simulink library "common_lib"  (R2023a)
settings: Solver=ode45  StartTime=0.0  StopTime=10.0  RelTol=1e-3
undefined symbols (not defined in the file): ACCEL_PRE_MULT, APDT_SrvcMgr_IRVHVDCSubFcnReq, C_C1GearNumbers, C_C1GearRatios, C_Calibration, C_DitherWaveform, C_GearOffset, C_GearRatioIn, C_GearRatioInverseOut, C_GearRatioOut, CLUTCH_INNER_LOOP_UPDATE_RATE, CONSTANT, DEGRADED_MODE_SIZE, Dem_EventStatusType, DiscIntNeverNeededParam, F_FAULT_ENUM, F_NOFAULT, F_OUTOFRANGE, F_RATELIMIT, FALSE, FMI14_SPECIAL_INSTRUCTIONS, FMI20_DATA_DRIFTED_HIGH, FMI21_DATA_DRIFTED_LOW, FMI29_RESERVED_FOR_SAE_ASSIGNMENT, FMI30_RESERVED_FOR_SAE_ASSIGNMENT, FMI31_CONDITION_EXISTS, FMI32_NO_FAULT, IC, k_accel, k_mean, MAX_UINT32, MEAN_PRE_MULT, NTriggers, QLTY_SIGNAL_FAILED, QLTY_SIGNAL_FULLY_FUNCTION, QLTY_SIGNAL_SUBSTITUTED_BY_1ST_CHOICE, QLTY_SIGNAL_SUBSTITUTED_BY_2ND_CHOICE, QLTY_SIGNAL_SUBSTITUTED_BY_3RD_CHOICE, QLTY_SIGNAL_SUBSTITUTED_BY_4TH_CHOICE, SAMPLE_TIME_100us, SAMPLETIME_10ms_Int, SATURATION_U16, simin, T_TestPoint, TF_FALSE, TF_TRUE, TimeStep, TRUE, WORKSPACE_UPDATE_RATE, ZERO, Zero
libraries: $bdroot x123, simulink x28, simulink_extras x4, MBD_EPS_Local_Blockset x4
(part 7 of 10)

== system common_lib/Gear Ratios/FindGearNumberByRatio ==
  note: If either the output speed, or the clutch speed is above minimum
      | then report that the speed is above minimum speed for detection.  However,
      | only output a gear other than zero to the GearNumber if OS > min speed.  This is done
      | because if the OS is stopped, but the clutch speed is still > min, you can tell
      | that there is no ratio being imposed.  So GearNumber should report zero, and the speeds are
      | above the threshold for detecting this condition.
  note: This block finds the gear number that corresponds to the ratio
      | between the os and clutch speed.  The output speed must be above the MinSpeed, and the ratio must be
      | within the SpeedTolerance for at least a time of ConfirmTime before OutputValid goes true.
      | If OutputValid is false then the GearNumber output does not have any meaning.
  OutputSpeed : Inport
  ClutchSpeed : Inport  Port=2
  SpeedTolerance : Inport  Port=3
  MinSpeed : Inport  Port=4
  Abs : Abs  ZeroCross=off  SaturateOnIntegerOverflow=off
  Abs1 : Abs  ZeroCross=off  SaturateOnIntegerOverflow=off
  Abs2 : Abs  ZeroCross=off  SaturateOnIntegerOverflow=off
  ClampAroundZero : $bdroot/Misc/ClampAroundZero  Tol=single(0.1)
      settings: AttributesFormatString=tol=%<Tol>
  Constant1 : Constant  Value=ConfirmTime
  Constant2 : Constant  Value=single(0)
  GearToRatio : Lookup  InputValues=GearToRatioIn  Table=GearToRatioOut  LookUpMeth=Use Input Nearest  SaturateOnIntegerOverflow=off
  Logical Operator : Logic  AllPortsSameDT=off
  Logical Operator1 : Logic  Operator=OR  AllPortsSameDT=off
  Product1 : Product  Inputs=/*  RndMeth=Zero
  Product2 : Product  Inputs=**  RndMeth=Zero
  RatioToGear : Lookup  InputValues=RatioToGearIn  Table=RatioToGearOut  LookUpMeth=Use Input Nearest  SaturateOnIntegerOverflow=off
  Relational Operator : RelationalOperator  Operator=<  ZeroCross=off  InputSameDT=off
  Relational Operator1 : RelationalOperator  Operator=>  ZeroCross=off  InputSameDT=off
  Relational Operator2 : RelationalOperator  Operator=>  ZeroCross=off  InputSameDT=off
  Sum : Sum  Inputs=-+
  Switch : Switch  Threshold=0.5  ZeroCross=off  SaturateOnIntegerOverflow=off  InputSameDT=off
  Timer1 : Subsystem  mask{TimeStep=0}
      mask prompts: TimeStep "Time Step (double)"
      mask help:
      | This block outputs a boolean true when In has been true
      | for at least the TiggerTime time.
  GearNumber : Outport  VectorParamsAs1DForOutWhenUnconnected=off
  OutputValid : Outport  Port=2  VectorParamsAs1DForOutWhenUnconnected=off
  SpeedAboveMin : Outport  Port=3  VectorParamsAs1DForOutWhenUnconnected=off
  wires:
  Relational Operator2/1 -> Logical Operator1/2
  Abs2/1 -> Relational Operator2/1
  Logical Operator1/1 -> SpeedAboveMin/1
  ClampAroundZero/1 -> Product1/1, Product2/2, Abs1/1
  Constant1/1 -> Timer1/2(TriggerTime)
  Timer1/1(Out) -> Switch/2, OutputValid/1
  Logical Operator/1 -> Timer1/1(In)
  Product1/1 -> RatioToGear/1
  ClutchSpeed/1 -> Abs2/1, Sum/2, Product1/2
  RatioToGear/1 -> GearToRatio/1, Switch/1  "nearest_gear_number"
  GearToRatio/1 -> Product2/1  "nearest_ratio"
  Product2/1 -> Sum/1  "nearest_speed_byratio"
  Abs/1 -> Relational Operator/1
  Sum/1 -> Abs/1
  SpeedTolerance/1 -> Relational Operator/2
  Relational Operator/1 -> Logical Operator/1
  Constant2/1 -> Switch/3
  OutputSpeed/1 -> ClampAroundZero/1
  Switch/1 -> GearNumber/1
  Abs1/1 -> Relational Operator1/1
  MinSpeed/1 -> Relational Operator2/2, Relational Operator1/2
  Relational Operator1/1 -> Logical Operator1/1, Logical Operator/2

== system common_lib/Gear Ratios/GearNumberToRatio ==
  gear_number : Inport
  C_GearInverseRatio : LookupNDDirect  NumberOfTableDimensions=1  Table=C_GearRatioInverseOut
  C_GearRatio : LookupNDDirect  NumberOfTableDimensions=1  Table=C_GearRatioOut
  Constant5 : Constant  Value=int8(-99)  SampleTime=-1
  GearOffset : Constant  Value=C_GearOffset  SampleTime=-1
  GearOffset1 : Constant  Value=int8(0)  SampleTime=-1
  Relational Operator3 : RelationalOperator  Operator=~=  ZeroCross=off
  Subtract : Sum
  Switch : Switch  Threshold=0.5  ZeroCross=off  SaturateOnIntegerOverflow=off  InputSameDT=off
  ratio : Outport  VectorParamsAs1DForOutWhenUnconnected=off
  inv_ratio : Outport  Port=2  VectorParamsAs1DForOutWhenUnconnected=off
  wires:
  GearOffset1/1 -> Switch/3
  Relational Operator3/1 -> Switch/2
  Constant5/1 -> Relational Operator3/2
  GearOffset/1 -> Subtract/2
  Subtract/1 -> C_GearRatio/1, C_GearInverseRatio/1
  Switch/1 -> Subtract/1
  gear_number/1 -> Switch/1, Relational Operator3/1
  C_GearRatio/1 -> ratio/1
  C_GearInverseRatio/1 -> inv_ratio/1

== system common_lib/IO/Calibration with Pretty Print Value ==
  C_Calibration : Constant  Value=CalValue  SampleTime=-1
  Outport : Outport  VectorParamsAs1DForOutWhenUnconnected=off
  wires:
  C_Calibration/1 -> Outport/1

== system common_lib/IO/From Workspace w//Datatype ==
  Data Type Conversion : DataTypeConversion  SaturateOnIntegerOverflow=off  RndMeth=Floor
  From Workspace : FromWorkspace  VariableName=var  SampleTime=st  ZeroCross=off
  Out1 : Outport  VectorParamsAs1DForOutWhenUnconnected=off
  wires:
  From Workspace/1 -> Data Type Conversion/1
  Data Type Conversion/1 -> Out1/1

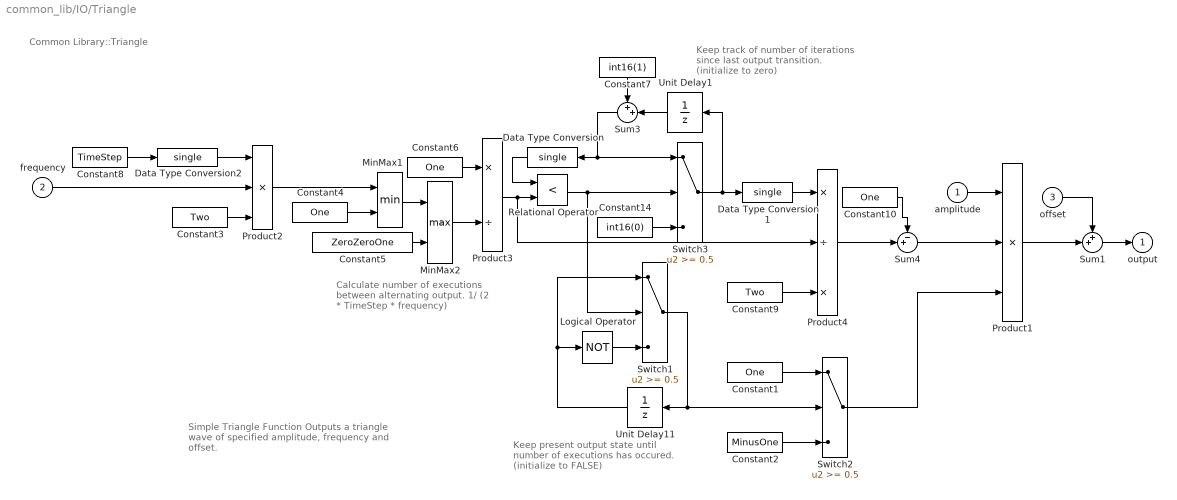
== system common_lib/IO/Triangle ==
  note: Common Library::Triangle
  note: Simple Triangle Function
      | Outputs a triangle wave of specified
      | amplitude, frequency and offset.
  note: Calculate number of executions
      | between alternating output.
      | 1/ (2 * TimeStep * frequency)
  note: Keep track of number of iterations
      | since last output transition.
      | (initialize to zero)
  note: Keep present output state until
      | number of executions has occured.
      | (initialize to FALSE)
  amplitude : Inport
  frequency : Inport  Port=2
  offset : Inport  Port=3
  Constant{1,4,6,10} (4 alike) : Constant  Value=One
  Constant14 : Constant  Value=int16(0)
  Constant2 : Constant  Value=MinusOne
  Constant3 : Constant  Value=Two
  Constant5 : Constant  Value=ZeroZeroOne
  Constant7 : Constant  Value=int16(1)
  Constant8 : Constant  Value=TimeStep
  Constant9 : Constant  Value=Two
  Data Type Conversion : DataTypeConversion  OutDataTypeStr=single  SaturateOnIntegerOverflow=off
  Data Type Conversion1 : DataTypeConversion  OutDataTypeStr=single  SaturateOnIntegerOverflow=off
  Data Type Conversion2 : DataTypeConversion  OutDataTypeStr=single  SaturateOnIntegerOverflow=off  RndMeth=Floor
  Logical Operator : Logic  Operator=NOT
  MinMax1 : MinMax  Inputs=2  InputSameDT=on  SaturateOnIntegerOverflow=on  ZeroCross=off
  MinMax2 : MinMax  Function=max  Inputs=2  InputSameDT=on  SaturateOnIntegerOverflow=on  ZeroCross=off
  Product1 : Product  Inputs=3  InputSameDT=on  OutDataTypeStr=Inherit: Same as first input
  Product2 : Product  Inputs=***  InputSameDT=on  OutDataTypeStr=Inherit: Same as first input
  Product3 : Product  Inputs=*/  InputSameDT=on  OutDataTypeStr=Inherit: Same as first input
  Product4 : Product  Inputs=*/*  InputSameDT=on  OutDataTypeStr=Inherit: Same as first input
  Relational Operator : RelationalOperator  Operator=<  ZeroCross=off
  Sum1 : Sum  Inputs=++|  InputSameDT=on  OutDataTypeStr=Inherit: Same as first input
  Sum3 : Sum  Inputs=++|  InputSameDT=on  OutDataTypeStr=Inherit: Same as first input
  Sum4 : Sum  Inputs=-+|  InputSameDT=on  OutDataTypeStr=Inherit: Same as first input
  Switch1 : Switch  Threshold=0.5  ZeroCross=off  SaturateOnIntegerOverflow=off
  Switch2 : Switch  Threshold=0.5  ZeroCross=off  SaturateOnIntegerOverflow=off
  Switch3 : Switch  Threshold=0.5  ZeroCross=off  SaturateOnIntegerOverflow=off
  Unit Delay1 : UnitDelay  SampleTime=-1  HasFrameUpgradeWarning=on
  Unit Delay11 : UnitDelay  InitialCondition=false  SampleTime=-1  HasFrameUpgradeWarning=on
  output : Outport  VectorParamsAs1DForOutWhenUnconnected=off
  wires:
  Constant8/1 -> Data Type Conversion2/1
  Data Type Conversion2/1 -> Product2/1
  Switch2/1 -> Product1/3
  Constant2/1 -> Switch2/3
  Constant1/1 -> Switch2/1
  Sum4/1 -> Product1/2
  Product4/1 -> Sum4/2
  Constant10/1 -> Sum4/1
  Constant9/1 -> Product4/3
  Data Type Conversion1/1 -> Product4/1
  offset/1 -> Sum1/1
  Unit Delay11/1 -> Logical Operator/1, Switch1/1
  Switch1/1 -> Switch2/2, Unit Delay11/1
  Product1/1 -> Sum1/2
  amplitude/1 -> Product1/1
  frequency/1 -> Product2/2
  Product2/1 -> MinMax1/1
  Constant4/1 -> MinMax1/2
  MinMax1/1 -> MinMax2/1
  Constant5/1 -> MinMax2/2
  Sum1/1 -> output/1
  MinMax2/1 -> Product3/2
  Constant6/1 -> Product3/1
  Constant3/1 -> Product2/3
  Switch3/1 -> Data Type Conversion1/1, Unit Delay1/1
  Constant14/1 -> Switch3/3
  Unit Delay1/1 -> Sum3/2
  Constant7/1 -> Sum3/1
  Sum3/1 -> Switch3/1, Data Type Conversion/1
  Logical Operator/1 -> Switch1/3
  Product3/1 -> Product4/2, Relational Operator/2
  Relational Operator/1 -> Switch3/2, Switch1/2
  Data Type Conversion/1 -> Relational Operator/1

== system common_lib/Integrators/ForwardEulerIntergrator ==
  dx : Inport
  x0 : Inport  Port=2
  reset : Inport  Port=3
  Constant2 : Constant  Value=TSAMP  SampleTime=-1
  Data Type Conversion : DataTypeConversion  OutDataTypeStr=single  SaturateOnIntegerOverflow=off
  Divide : Product  Inputs=**
  Sum : Sum  Inputs=|++
  Switch1 : Switch  Threshold=0.5  ZeroCross=off  SaturateOnIntegerOverflow=off  InputSameDT=off
  Unit Delay : UnitDelay  InitialCondition=IC  SampleTime=-1  HasFrameUpgradeWarning=on
      settings: AttributesFormatString=ic=%<X0>
  x : Outport  VectorParamsAs1DForOutWhenUnconnected=off
  wires:
  Data Type Conversion/1 -> Divide/2
  Sum/1 -> Unit Delay/1
  Unit Delay/1 -> Switch1/3
  Switch1/1 -> x/1, Sum/2
  x0/1 -> Switch1/1
  reset/1 -> Switch1/2
  dx/1 -> Divide/1
  Divide/1 -> Sum/1
  Constant2/1 -> Data Type Conversion/1

== system common_lib/Misc/ArcSine ==
  note: Common Library::Trigonometry:Sine
  note: Taylor Series Expansion for ArcSIN
      | Best Accuracy from -pi/3 to +pi/3
  angle : Inport
  Constant5 : Constant  Value=single(1/6)
  Constant6 : Constant  Value=single(3/40)
  Constant7 : Constant  Value=single(15/336)
  Constant9 : Constant  Value=single(105/3456)
  Product{1..2,4..5} (4 alike) : Product  OutDataTypeStr=Inherit: Same as first input
  Product{3,6..8} (4 alike) : Product  Inputs=3  OutDataTypeStr=Inherit: Same as first input
  Sum1 : Sum  Inputs=5
  asin : Outport  VectorParamsAs1DForOutWhenUnconnected=off
  wires:
  Sum1/1 -> asin/1
  Product6/1 -> Product4/1
  Product4/1 -> Sum1/5
  angle/1 -> Product7/2, Sum1/1, Product8/1, Product8/2, Product8/3, Product7/3, Product3/2, Product3/3, Product6/3, Product6/2
  Constant9/1 -> Product4/2
  Product2/1 -> Sum1/4
  Constant7/1 -> Product2/2
  Product3/1 -> Product2/1, Product6/1
  Product1/1 -> Sum1/3
  Constant6/1 -> Product1/2
  Product7/1 -> Product1/1, Product3/1
  Product5/1 -> Sum1/2
  Constant5/1 -> Product5/2
  Product8/1 -> Product7/1, Product5/1

== system common_lib/Misc/ClampAboveZero ==
  note: Common Library::Miscellaneous Computations::Clamp Above Zero
  input : Inport
  Constant : Constant  Value=Tol
  MinMax : MinMax  Function=max  Inputs=2  InputSameDT=on  SaturateOnIntegerOverflow=on  ZeroCross=off
  output : Outport  VectorParamsAs1DForOutWhenUnconnected=off
  wires:
  input/1 -> MinMax/1
  MinMax/1 -> output/1
  Constant/1 -> MinMax/2

== system common_lib/Misc/ClampAroundZero ==
  note: Common Library::Miscellaneous Computations::Clamp Around Zero
  input : Inport
  Abs : Abs  ZeroCross=off  SaturateOnIntegerOverflow=off
  Constant : Constant  Value=Tol
  Constant1 : Constant  Value=Zero
  Constant2 : Constant  Value=One
  Constant3 : Constant  Value=MinusOne
  MinMax : MinMax  Function=max  Inputs=2  InputSameDT=on  SaturateOnIntegerOverflow=on  ZeroCross=off
  Product : Product  InputSameDT=on  OutDataTypeStr=Inherit: Same as first input
  Relational Operator : RelationalOperator  ZeroCross=off
  Switch1 : Switch  Threshold=0.5  ZeroCross=off  SaturateOnIntegerOverflow=off
  output : Outport  VectorParamsAs1DForOutWhenUnconnected=off
  wires:
  Constant/1 -> MinMax/2
  Abs/1 -> MinMax/1
  input/1 -> Abs/1, Relational Operator/1
  MinMax/1 -> Product/2
  Switch1/1 -> Product/1
  Product/1 -> output/1
  Constant1/1 -> Relational Operator/2
  Relational Operator/1 -> Switch1/2
  Constant2/1 -> Switch1/1
  Constant3/1 -> Switch1/3

== system common_lib/Misc/Cosine ==
  note: Taylor Series Expansion for COS(x)
  note: Common Library::Trigonometry:Cosine
  angle : Inport
  Constant : Constant  Value=single(1/(1*2))
  Constant1 : Constant  Value=single(1/(1*2*3*4))
  Constant2 : Constant  Value=single(1)
  Product : Product  OutDataTypeStr=Inherit: Same as first input
  Product1 : Product  OutDataTypeStr=Inherit: Same as first input
  Product3 : Product  OutDataTypeStr=Inherit: Same as first input
  Product6 : Product  Inputs=3  OutDataTypeStr=Inherit: Same as first input
  Sum : Sum  Inputs=+-+
  cos : Outport  VectorParamsAs1DForOutWhenUnconnected=off
  wires:
  Product/1 -> Sum/2
  Product1/1 -> Sum/3
  Sum/1 -> cos/1
  angle/1 -> Product3/2, Product6/2, Product6/3, Product3/1
  Product3/1 -> Product6/1, Product/1
  Constant1/1 -> Product1/2
  Constant/1 -> Product/2
  Product6/1 -> Product1/1
  Constant2/1 -> Sum/1

== system common_lib/Misc/Count Edges ==
  note: Common Library::Miscellaneous::Count Edges
  Input : Inport
  Reset : Inport  Port=2
  Logical Operator5 : Logic  Operator=NOT  AllPortsSameDT=off
  Logical Operator6 : Logic  AllPortsSameDT=off
  Sum : Sum  Inputs=|++  InputSameDT=on  OutDataTypeStr=Inherit: Same as first input
  Switch1 : Switch  Threshold=0.5  ZeroCross=off  SaturateOnIntegerOverflow=off  InputSameDT=off
  Switch2 : Switch  Threshold=0.5  ZeroCross=off  SaturateOnIntegerOverflow=off  InputSameDT=off
  Unit Delay2 : UnitDelay  InitialCondition=int8(0)  SampleTime=-1  HasFrameUpgradeWarning=on
      settings: AttributesFormatString=ic=%<X0>
  Unit Delay3 : UnitDelay  InitialCondition=true  SampleTime=-1  HasFrameUpgradeWarning=on
      settings: AttributesFormatString=ic=%<X0>
  constant7 : Constant  Value=int8(0)
  constant8 : Constant  Value=int8(1)
  constant9 : Constant  Value=int8(0)
  Count : Outport  VectorParamsAs1DForOutWhenUnconnected=off
  wires:
  Reset/1 -> Switch1/2
  Input/1 -> Logical Operator6/1, Unit Delay3/1
  Switch1/1 -> Sum/2
  Unit Delay2/1 -> Count/1, Switch1/3
  constant9/1 -> Switch1/1
  Switch2/1 -> Sum/1
  Logical Operator6/1 -> Switch2/2
  Logical Operator5/1 -> Logical Operator6/2
  Unit Delay3/1 -> Logical Operator5/1
  constant8/1 -> Switch2/1
  constant7/1 -> Switch2/3
  Sum/1 -> Unit Delay2/1

== system common_lib/Misc/Count to X ==
  note: Common Library::Miscellaneous::Count to X
  input : Inport
  reset? : Inport  Port=2
  Constant1 : Constant  Value=uint8(1)
  Constant2 : Constant  Value=uint8(0)
  Constant3 : Constant  Value=uint8(X)
  Constant4 : Constant  Value=uint8(0)
  DelayedInput : Logic  Operator=NAND
  Input : Logic
  Logical Operator8 : Logic
  MinMax : MinMax  Inputs=2  InputSameDT=on  SaturateOnIntegerOverflow=on  ZeroCross=off
  Relational Operator : RelationalOperator  ZeroCross=off
  Sum1 : Sum  Inputs=++|  InputSameDT=on  OutDataTypeStr=Inherit: Same as first input
  Unit Delay : UnitDelay  InitialCondition=uint8(0)  SampleTime=-1  HasFrameUpgradeWarning=on
  Unit Delay2 : UnitDelay  InitialCondition=false  SampleTime=-1  HasFrameUpgradeWarning=on
  inc switch : Switch  Threshold=0.5  ZeroCross=off  SaturateOnIntegerOverflow=off
  reset switch : Switch  Threshold=0.5  ZeroCross=off  SaturateOnIntegerOverflow=off
  output : Outport  VectorParamsAs1DForOutWhenUnconnected=off
  wires:
  Relational Operator/1 -> output/1
  Constant3/1 -> Relational Operator/2, MinMax/1
  Constant2/1 -> inc switch/3
  Constant1/1 -> inc switch/1
  Constant4/1 -> reset switch/1
  input/1 -> Unit Delay2/1, Input/1, Input/2
  Input/1 -> Logical Operator8/1
  Unit Delay2/1 -> DelayedInput/1, DelayedInput/2
  DelayedInput/1 -> Logical Operator8/2
  inc switch/1 -> Sum1/2
  Logical Operator8/1 -> inc switch/2
  Sum1/1 -> Relational Operator/1, MinMax/2
  reset switch/1 -> Sum1/1
  Unit Delay/1 -> reset switch/3
  reset?/1 -> reset switch/2
  MinMax/1 -> Unit Delay/1

== system common_lib/Misc/Counter ==
  note: Counter increments when "incr condition" is TRUE and decrements when "decr condition" is TRUE.
  note: Common Library::Miscellaneous::Counter
  up_val : Inport
  count_up? : Inport  Port=2  OutDataTypeStr=boolean
  down_val : Inport  Port=3
  count_down? : Inport  Port=4  OutDataTypeStr=boolean
  max_count : Inport  Port=5
  min_count : Inport  Port=6
  reset? : Inport  Port=7  OutDataTypeStr=boolean
  Constant1 : Constant  Value=Zero
  Constant2 : Constant  Value=Zero
  Constant4 : Constant  Value=IC
  Constant5 : Constant  Value=false
  Logical Operator : Logic  Operator=OR
  Sat : $bdroot/Slink/Sat
  Sum : Sum  Inputs=++-  InputSameDT=on  OutDataTypeStr=Inherit: Same as first input
  Unit Delay : UnitDelay  InitialCondition=IC  SampleTime=-1  HasFrameUpgradeWarning=on
  Unit Delay1 : UnitDelay  InitialCondition=true  SampleTime=-1  HasFrameUpgradeWarning=on
  dec switch : Switch  Threshold=0.5  ZeroCross=off  SaturateOnIntegerOverflow=off
  inc switch : Switch  Threshold=0.5  ZeroCross=off  SaturateOnIntegerOverflow=off
  reset switch : Switch  Threshold=0.5  ZeroCross=off  SaturateOnIntegerOverflow=off
  output : Outport  VectorParamsAs1DForOutWhenUnconnected=off
  wires:
  count_down?/1 -> dec switch/2
  down_val/1 -> dec switch/1
  count_up?/1 -> inc switch/2
  up_val/1 -> inc switch/1
  Constant2/1 -> dec switch/3
  dec switch/1 -> Sum/3
  Constant1/1 -> inc switch/3
  inc switch/1 -> Sum/2
  reset?/1 -> Logical Operator/1
  reset switch/1 -> Unit Delay/1, output/1
  Unit Delay/1 -> Sum/1
  Logical Operator/1 -> reset switch/2
  Unit Delay1/1 -> Logical Operator/2
  Constant5/1 -> Unit Delay1/1
  Sat/1 -> reset switch/3
  Constant4/1 -> reset switch/1
  max_count/1 -> Sat/2
  min_count/1 -> Sat/3
  Sum/1 -> Sat/1

== system common_lib/Misc/Divide by X ==
  note: Common Library::Miscellaneous::Divide by X
  trigger? : Inport
  Constant1 : Constant  Value=uint8(X)
  Constant2 : Constant  Value=uint8(1)
  Constant3 : Constant  Value=uint8(X)
  Constant4 : Constant  Value=uint8(0)
  Relational Operator : RelationalOperator  ZeroCross=off
  Sum1 : Sum  Inputs=|++  InputSameDT=on  OutDataTypeStr=Inherit: Same as first input
  Unit Delay : UnitDelay  InitialCondition=uint8(X)  SampleTime=-1  HasFrameUpgradeWarning=on
  inc switch : Switch  Threshold=0.5  ZeroCross=off  SaturateOnIntegerOverflow=off
  reset switch : Switch  Threshold=0.5  ZeroCross=off  SaturateOnIntegerOverflow=off
  output : Outport  VectorParamsAs1DForOutWhenUnconnected=off
  wires:
  Constant4/1 -> reset switch/1
  Constant1/1 -> inc switch/1
  Constant2/1 -> Sum1/1
  trigger?/1 -> inc switch/2
  Sum1/1 -> inc switch/3
  inc switch/1 -> Relational Operator/1, reset switch/3
  Constant3/1 -> Relational Operator/2
  Unit Delay/1 -> Sum1/2
  Relational Operator/1 -> reset switch/2, output/1
  reset switch/1 -> Unit Delay/1

== system common_lib/Misc/EatonLogo ==

== system common_lib/Misc/EdgeTriggered Pulse ==
  note: Common Library::Miscellaneous::Edge Triggered Pulse
  input : Inport
  ETP : $bdroot/Misc/EdgeTriggered Pulse w time  Edge=TRUE to FALSE  Pulse=TRUE  TimeStep=[]  Init=0
  Timeout Threshold : Constant  Value=Width
  pulse : Outport  VectorParamsAs1DForOutWhenUnconnected=off
  wires:
  input/1 -> ETP/1
  Timeout Threshold/1 -> ETP/2
  ETP/1 -> pulse/1

== system common_lib/Misc/EdgeTriggered Pulse w time ==
  note: 0 = PULSE_FALSE
      | 1 = PULSE_TRUE
  note: 0 = FALSE_TO_TRUE
      | 1 = TRUE_TO_FALSE
  input : Inport  OutDataTypeStr=boolean
  width : Inport  Port=2  OutDataTypeStr=single
  Data Type Conversion : DataTypeConversion  OutDataTypeStr=single  RndMeth=Floor
  EdgeTriggeredPulseCoreLogic : Subsystem  TreatAsAtomicUnit=on  RTWFcnName=ETPWT
      settings: RTWSystemCode=Inline  RTWFcnNameOpts=User specified  RTWFileNameOpts=Use function name
  Output : Constant  Value=OUTPUT
  Trigger : Constant  Value=TRIGGER
  XOR_IN : Logic  Operator=XOR
  XOR_OUT : Logic  Operator=XOR
  pulse : Outport  OutDataTypeStr=boolean  VectorParamsAs1DForOutWhenUnconnected=off
  wires:
  XOR_IN/1 -> EdgeTriggeredPulseCoreLogic/1(input)
  width/1 -> Data Type Conversion/1
  Output/1 -> XOR_OUT/1
  EdgeTriggeredPulseCoreLogic/1(pulse) -> XOR_OUT/2
  XOR_OUT/1 -> pulse/1
  input/1 -> XOR_IN/2
  Trigger/1 -> XOR_IN/1
  Data Type Conversion/1 -> EdgeTriggeredPulseCoreLogic/2(width)

== system common_lib/Misc/GreenLeaf_Globe ==

== system common_lib/Misc/Hold ==
  in : Inport
  Enable : EnablePort  ZeroCross=off
  out : Outport  VectorParamsAs1DForOutWhenUnconnected=off
  wires:
  in/1 -> out/1

== system common_lib/Misc/Latch ==
  note: Output signal is latched to true until reset input is true.
  note: Common Library::Miscellaneous::Latch
  input : Inport  OutDataTypeStr=boolean
  reset? : Inport  Port=2  OutDataTypeStr=boolean
  Constant2 : Constant  Value=false
  Constant3 : Constant  Value=true
  Switch : Switch  Threshold=0.5  ZeroCross=off
  Switch1 : Switch  Threshold=0.5  ZeroCross=off
  Unit Delay1 : UnitDelay  InitialCondition=IC  SampleTime=-1  HasFrameUpgradeWarning=on
  output : Outport  VectorParamsAs1DForOutWhenUnconnected=off
  wires:
  Switch/1 -> Unit Delay1/1, output/1
  reset?/1 -> Switch/2
  Constant2/1 -> Switch/1
  Switch1/1 -> Switch/3
  Unit Delay1/1 -> Switch1/3
  input/1 -> Switch1/2
  Constant3/1 -> Switch1/1

== system common_lib/Misc/ModelVersion ==
  Terminator : Terminator
  mdlVersionBlock : Constant  Value=mdlVersion  SampleTime=-1
  wires:
  mdlVersionBlock/1 -> Terminator/1  "DiagBusVolt_SwcVer"

== system common_lib/Misc/NonZero ==
  InputValue : Inport
  Abs : Abs  ZeroCross=off
  Constant : Constant  Value=Tol
  Relational Operator : RelationalOperator  ZeroCross=off  InputSameDT=off
  SrvcMgr_IGBTSrvcIGBT6Offset : Outport  InitialOutput=APDT_SrvcMgr_IRVHVDCSubFcnReq.SrvcMgr_IRVHVDCSubFcnReq_NoReq  VectorParamsAs1DForOutWhenUnconnected=off
  wires:
  InputValue/1 -> Abs/1
  Relational Operator/1 -> SrvcMgr_IGBTSrvcIGBT6Offset/1
  Constant/1 -> Relational Operator/2
  Abs/1 -> Relational Operator/1

== system common_lib/Misc/Sine ==
  note: Taylor Series Expansion for SIN(x)
  note: Common Library::Trigonometry:Sine
  angle : Inport
  Constant : Constant  Value=single(1/(1*2*3))
  Constant1 : Constant  Value=single(1/(1*2*3*4*5))
  Product : Product  OutDataTypeStr=Inherit: Same as first input
  Product1 : Product  OutDataTypeStr=Inherit: Same as first input
  Product3 : Product  Inputs=3  OutDataTypeStr=Inherit: Same as first input
  Product6 : Product  Inputs=3  OutDataTypeStr=Inherit: Same as first input
  Sum : Sum  Inputs=+-+
  sin : Outport  VectorParamsAs1DForOutWhenUnconnected=off
  wires:
  Product/1 -> Sum/2
  Product1/1 -> Sum/3
  Sum/1 -> sin/1
  angle/1 -> Product6/3, Product6/2, Product3/3, Product3/2, Product3/1, Sum/1
  Product3/1 -> Product6/1, Product/1
  Constant1/1 -> Product1/2
  Constant/1 -> Product/2
  Product6/1 -> Product1/1

== system common_lib/Misc/Tangent ==
  note: Taylor Series Expansion for TAN(x)
  note: Common Library::Trigonometry::Tangent
  angle : Inport
  Constant : Constant  Value=single(1/3)
  Constant1 : Constant  Value=single(2/15)
  Product1 : Product  Inputs=3  OutDataTypeStr=Inherit: Same as first input
  Product3 : Product  OutDataTypeStr=Inherit: Same as first input
  Product4 : Product  OutDataTypeStr=Inherit: Same as first input
  Product6 : Product  Inputs=3  OutDataTypeStr=Inherit: Same as first input
  Sum : Sum  Inputs=+++
  tan : Outport  VectorParamsAs1DForOutWhenUnconnected=off
  wires:
  Product4/1 -> Sum/3
  Product3/1 -> Sum/2
  Constant/1 -> Product3/2
  angle/1 -> Sum/1, Product1/1, Product1/2, Product1/3, Product6/2, Product6/3
  Sum/1 -> tan/1
  Constant1/1 -> Product4/2
  Product1/1 -> Product3/1, Product6/1
  Product6/1 -> Product4/1

== system common_lib/Misc/Timeout Detection ==
  note: Common Library::Miscellaneous::Timeout Detection
  value : Inport
  Data Type Conversion : DataTypeConversion  OutDataTypeStr=single  SaturateOnIntegerOverflow=off  RndMeth=Floor
  Relational Operator : RelationalOperator  Operator===  OutDataTypeStr=boolean  ZeroCross=off
  Relational Operator1 : RelationalOperator  Operator=>  OutDataTypeStr=boolean  ZeroCross=off
  Timeout Threshold : Constant  Value=Timeout
  TimeoutLogic : Subsystem  TreatAsAtomicUnit=on  RTWFcnName=TIMEOUT
      settings: RTWSystemCode=Inline  RTWFcnNameOpts=User specified  RTWFileNameOpts=Use function name
  Unit Delay1 : UnitDelay  InitialCondition=Zero  SampleTime=-1  HasFrameUpgradeWarning=on
  timeout? : Outport  VectorParamsAs1DForOutWhenUnconnected=off
  wires:
  TimeoutLogic/1(time) -> Relational Operator1/1
  Timeout Threshold/1 -> Data Type Conversion/1
  Relational Operator1/1 -> timeout?/1
  Unit Delay1/1 -> Relational Operator/2
  Relational Operator/1 -> TimeoutLogic/1(Change)
  value/1 -> Unit Delay1/1, Relational Operator/1
  Data Type Conversion/1 -> Relational Operator1/2, TimeoutLogic/2(Timeout)

== system common_lib/Misc/Timeout with time ==
  note: Common Library::Miscellaneous::Timeout Detection
  value : Inport
  timeout : Inport  Port=2
  Data Type Conversion : DataTypeConversion  OutDataTypeStr=single  RndMeth=Floor
  Relational Operator : RelationalOperator  Operator===  OutDataTypeStr=boolean  ZeroCross=off
  Relational Operator1 : RelationalOperator  Operator=>  OutDataTypeStr=boolean  ZeroCross=off
  TimeoutLogic : Subsystem  TreatAsAtomicUnit=on  RTWFcnName=TIMEOUT
      settings: RTWSystemCode=Inline  RTWFcnNameOpts=User specified  RTWFileNameOpts=Use function name
  Unit Delay1 : UnitDelay  InitialCondition=Zero  SampleTime=-1  HasFrameUpgradeWarning=on
  timeout? : Outport  VectorParamsAs1DForOutWhenUnconnected=off
  wires:
  Data Type Conversion/1 -> TimeoutLogic/2(Timeout), Relational Operator1/2
  value/1 -> Relational Operator/1, Unit Delay1/1
  Relational Operator/1 -> TimeoutLogic/1(Change)
  Unit Delay1/1 -> Relational Operator/2
  Relational Operator1/1 -> timeout?/1
  timeout/1 -> Data Type Conversion/1
  TimeoutLogic/1(time) -> Relational Operator1/1

== system common_lib/Misc/Timeout with time Integer ==
  note: Common Library::Miscellaneous::Timeout Detection
  value : Inport
  timeout : Inport  Port=2
  Relational Operator : RelationalOperator  Operator===  OutDataTypeStr=boolean  ZeroCross=off
  Relational Operator1 : RelationalOperator  Operator=>  OutDataTypeStr=boolean  ZeroCross=off
  TimeoutLogic : Subsystem  TreatAsAtomicUnit=on  RTWFcnName=TIMEOUT
      settings: RTWSystemCode=Inline  RTWFcnNameOpts=User specified  RTWFileNameOpts=Use function name
  Unit Delay1 : UnitDelay  InitialCondition=Zero  SampleTime=-1  HasFrameUpgradeWarning=on
  timeout? : Outport  VectorParamsAs1DForOutWhenUnconnected=off
  wires:
  TimeoutLogic/1(time) -> Relational Operator1/1
  Relational Operator1/1 -> timeout?/1
  Unit Delay1/1 -> Relational Operator/2
  Relational Operator/1 -> TimeoutLogic/1(Change)
  value/1 -> Unit Delay1/1, Relational Operator/1
  timeout/1 -> Relational Operator1/2, TimeoutLogic/2(Timeout)

== system common_lib/Misc/Value Latch1 ==
  note: Common Library::Miscellaneous::Latch
  input : Inport
  Switch : Switch  Threshold=0.5  ZeroCross=off  SaturateOnIntegerOverflow=off
  Timeout Detection : $bdroot/Misc/Timeout Detection  Timeout=HoldTime  TimeStep=TimeStep
  Unit Delay : UnitDelay  InitialCondition=IC  SampleTime=-1  HasFrameUpgradeWarning=on
      settings: AttributesFormatString=ic=%<X0>
  Unit Delay1 : UnitDelay  InitialCondition=TRUE  SampleTime=-1  HasFrameUpgradeWarning=on
      settings: AttributesFormatString=ic=%<X0>
  output : Outport  InitialOutput=0  VectorParamsAs1DForOutWhenUnconnected=off
  wires:
  Unit Delay1/1 -> Timeout Detection/1
  Timeout Detection/1 -> Switch/2, Unit Delay1/1
  Unit Delay/1 -> Switch/3
  input/1 -> Switch/1
  Switch/1 -> Unit Delay/1, output/1

== system common_lib/OS/Scheduler ==
  Interrupt : TriggerPort  TriggerType=function-call  VariantControl=(inherit)  StatesWhenEnabling=reset  ZeroCross=off
  Demux : Demux  Outputs=5
      settings: DisplayOption=none
  Function-Call Generator : simulink/Ports & Subsystems/Function-Call Generator  sample_time=-1  numberOfIterations=1  DisallowWideOutput=off
  Task 1 : Outport  VectorParamsAs1DForOutWhenUnconnected=off
  Task 2 : Outport  Port=2  VectorParamsAs1DForOutWhenUnconnected=off
  Task 3 : Outport  Port=3  VectorParamsAs1DForOutWhenUnconnected=off
  Task 4 : Outport  Port=4  VectorParamsAs1DForOutWhenUnconnected=off
  Task 5 : Outport  Port=5  VectorParamsAs1DForOutWhenUnconnected=off
  wires:
  Function-Call Generator/1 -> Demux/1
  Demux/1 -> Task 1/1
  Demux/2 -> Task 2/1
  Demux/3 -> Task 3/1
  Demux/4 -> Task 4/1
  Demux/5 -> Task 5/1

== system common_lib/OS/Scheduler with Init ==
  Interrupt : TriggerPort  TriggerType=function-call  VariantControl=(inherit)  StatesWhenEnabling=reset  ZeroCross=off
  Demux : Demux  Outputs=3
      settings: DisplayOption=none
  Function-Call Generator : simulink/Ports & Subsystems/Function-Call Generator  sample_time=-1  numberOfIterations=1  DisallowWideOutput=off
  Init Relay : Subsystem
  Init : Outport  VectorParamsAs1DForOutWhenUnconnected=off
  Task 1 : Outport  Port=2  VectorParamsAs1DForOutWhenUnconnected=off
  Task 2 : Outport  Port=3  VectorParamsAs1DForOutWhenUnconnected=off
  wires:
  Demux/3 -> Task 2/1
  Demux/2 -> Task 1/1
  Demux/1 -> Init Relay/Trigger
  Init Relay/1(Init) -> Init/1
  Function-Call Generator/1 -> Demux/1

== system common_lib/OS/fcn_call generator ==
  note: This component is an atomic element used by the
      | schedule_morph script to build scheduler blocks
  note: Common Library::OS::Function Call Generator
  Enable : EnablePort  StatesWhenEnabling=reset  ZeroCross=off
  Function-Call Generator : simulink/Ports & Subsystems/Function-Call Generator  sample_time=-1  numberOfIterations=1  DisallowWideOutput=off
  Out : Outport  VectorParamsAs1DForOutWhenUnconnected=off
  wires:
  Function-Call Generator/1 -> Out/1

== system common_lib/OS/schedule counter ==
  note: This component is an atomic element used by the
      | schedule_morph script to build scheduler blocks
  note: Common Library::OS::Schedule Counter
  Constant2 : Constant  Value=int8(1)
  Constant3 : Constant  Value=int8(1)
  Constant4 : Constant  Value=FALSE
  Constant5 : Constant  Value=int8(1)
  Logical Operator : Logic  Operator=OR
  MinMax1 : MinMax  Inputs=2  InputSameDT=on  ZeroCross=off
  NTriggers : Constant  Value=NTriggers
  Relational Operator1 : RelationalOperator  Operator=>  ZeroCross=off  InputSameDT=off
  Sum : Sum  Inputs=++|  InputSameDT=on  OutDataTypeStr=Inherit: Same as first input
  Sum1 : Sum  Inputs=|-+  InputSameDT=on  OutDataTypeStr=Inherit: Same as first input
  Unit Delay : UnitDelay  InitialCondition=int8(1)  SampleTime=-1  HasFrameUpgradeWarning=on
  Unit Delay1 : UnitDelay  InitialCondition=TRUE  SampleTime=-1  HasFrameUpgradeWarning=on
  reset switch : Switch  Threshold=0.5  ZeroCross=off  SaturateOnIntegerOverflow=off
  Counter : Outport  VectorParamsAs1DForOutWhenUnconnected=off
  wires:
  Constant5/1 -> Sum1/1
  Sum/1 -> MinMax1/2
  NTriggers/1 -> Sum1/2, MinMax1/1
  Sum1/1 -> Relational Operator1/2
  Relational Operator1/1 -> Logical Operator/1
  Constant3/1 -> reset switch/1
  MinMax1/1 -> reset switch/3
  Constant2/1 -> Sum/2
  Constant4/1 -> Unit Delay1/1
  Unit Delay1/1 -> Logical Operator/2
  Logical Operator/1 -> reset switch/2
  Unit Delay/1 -> Relational Operator1/1, Sum/1
  reset switch/1 -> Unit Delay/1, Counter/1

== system common_lib/OS/sequence generator ==
  note: This component is an atomic element used by the
      | schedule_morph script to build scheduler blocks
  note: Common Library::OS::Sequence Generator
  In : Inport
  Constant9 : Constant  Value=int8(1)
  Function-Call Generator : simulink/Ports & Subsystems/Function-Call Generator  sample_time=-1  numberOfIterations=1  DisallowWideOutput=off
  Sum1 : Sum  Inputs=|++  InputSameDT=on  OutDataTypeStr=Inherit: Same as first input
  Trigger : Outport  VectorParamsAs1DForOutWhenUnconnected=off
  Out : Outport  Port=2  VectorParamsAs1DForOutWhenUnconnected=off
  wires:
  Function-Call Generator/1 -> Trigger/1
  Constant9/1 -> Sum1/2
  In/1 -> Sum1/1
  Sum1/1 -> Out/1

== system common_lib/SCond/Gain and Offset (in) ==
  note: Common Library::Signal Conditioning::Gain and Offset (in)
  input : Inport
  gain : Inport  Port=2
  offset : Inport  Port=3
  InputConversion : DataTypeConversion  OutDataTypeStr=single  SaturateOnIntegerOverflow=off
  InputConversion1 : DataTypeConversion  OutDataTypeStr=single  SaturateOnIntegerOverflow=off
  InputConversion2 : DataTypeConversion  OutDataTypeStr=single  SaturateOnIntegerOverflow=off
  OutputConversion : DataTypeConversion  OutDataTypeStr=single  SaturateOnIntegerOverflow=off
  Product : Product  InputSameDT=on  OutDataTypeStr=Inherit: Same as first input
  Sum : Sum  Inputs=|+-  InputSameDT=on  OutDataTypeStr=Inherit: Same as first input
  output : Outport  VectorParamsAs1DForOutWhenUnconnected=off
  wires:
  OutputConversion/1 -> output/1
  input/1 -> InputConversion/1
  gain/1 -> InputConversion1/1
  Product/1 -> Sum/1
  offset/1 -> InputConversion2/1
  Sum/1 -> OutputConversion/1
  InputConversion/1 -> Product/1
  InputConversion1/1 -> Product/2
  InputConversion2/1 -> Sum/2

== system common_lib/SCond/Gain and Offset (out) ==
  note: Common Library::Signal Conditioning::Gain and Offset (out)
  input : Inport
  gain : Inport  Port=2
  offset : Inport  Port=3
  InputConversion : DataTypeConversion  OutDataTypeStr=single  SaturateOnIntegerOverflow=off
  InputConversion1 : DataTypeConversion  OutDataTypeStr=single  SaturateOnIntegerOverflow=off
  InputConversion2 : DataTypeConversion  OutDataTypeStr=single  SaturateOnIntegerOverflow=off
  OutputConversion : DataTypeConversion  OutDataTypeStr=single  SaturateOnIntegerOverflow=off
  Product : Product  Inputs=*/  InputSameDT=on  OutDataTypeStr=Inherit: Same as first input
  Sum : Sum  Inputs=|++  InputSameDT=on  OutDataTypeStr=Inherit: Same as first input
  output : Outport  VectorParamsAs1DForOutWhenUnconnected=off
  wires:
  Sum/1 -> Product/1
  input/1 -> InputConversion/1
  OutputConversion/1 -> output/1
  offset/1 -> InputConversion1/1
  gain/1 -> InputConversion2/1
  Product/1 -> OutputConversion/1
  InputConversion/1 -> Sum/1
  InputConversion1/1 -> Sum/2
  InputConversion2/1 -> Product/2

== system common_lib/SCond/Membership Function ==
  x : Inport
  Compare1 : RelationalOperator  Operator=<=  ZeroCross=off
  MinMax : MinMax  Function=max  Inputs=2  InputSameDT=on  SaturateOnIntegerOverflow=on  ZeroCross=off
  Product2 : Product  Inputs=**  OutDataTypeStr=Inherit: Same as first input
  Sum1 : Sum  Inputs=|++  InputSameDT=on  OutDataTypeStr=Inherit: Same as first input
  Sum2 : Sum  Inputs=-+|  InputSameDT=on  OutDataTypeStr=Inherit: Same as first input
  Switch1 : Switch  Criteria=u2 ~= 0  Threshold=0.5  ZeroCross=off  SaturateOnIntegerOverflow=off
  TRUE1 : Constant  Value=SlopeLow
  TRUE3 : Constant  Value=Peak
  TRUE4 : Constant  Value=One
  TRUE5 : Constant  Value=Zero
  TRUE6 : Constant  Value=SlopeHigh
  TRUE7 : Constant  Value=Peak
  mu(x) : Outport  VectorParamsAs1DForOutWhenUnconnected=off
  wires:
  Sum1/1 -> MinMax/2
  Switch1/1 -> Product2/2
  Product2/1 -> Sum1/1
  TRUE3/1 -> Compare1/2
  Compare1/1 -> Switch1/2
  TRUE6/1 -> Switch1/3
  TRUE1/1 -> Switch1/1
  Sum2/1 -> Product2/1
  TRUE7/1 -> Sum2/1
  x/1 -> Compare1/1, Sum2/2
  TRUE4/1 -> Sum1/2
  TRUE5/1 -> MinMax/1
  MinMax/1 -> mu(x)/1

== system common_lib/SCond/Test Override Gain and Offset (in) ==
  note: This block  accepts the Inputsignal, gain, offset, and override flag
      |
      | This block does the  functionality of Y =mX+b
      | Where  Y  = Output
      |               m = Override_Gain
      |               X  = Input
      |               b = Override_Offset
  note: Common Library::Signal Override::Gain , Offset ,Override flag
  Input : Inport
  Override_Gain : Inport  Port=2
  Override_Offset : Inport  Port=3
  Override_Flag : Inport  Port=4
  InputConversion : DataTypeConversion  OutDataTypeStr=single  SaturateOnIntegerOverflow=off
  InputConversion1 : DataTypeConversion  OutDataTypeStr=single  SaturateOnIntegerOverflow=off
  InputConversion2 : DataTypeConversion  OutDataTypeStr=single  SaturateOnIntegerOverflow=off
  OutputConversion : DataTypeConversion  OutDataTypeStr=single  SaturateOnIntegerOverflow=off
  Product : Product  InputSameDT=on  OutDataTypeStr=Inherit: Same as first input
  Sum : Sum  Inputs=|++  InputSameDT=on  OutDataTypeStr=Inherit: Same as first input
  Switch : Switch  Threshold=0.5  ZeroCross=off  SaturateOnIntegerOverflow=off  InputSameDT=off
  Output : Outport  VectorParamsAs1DForOutWhenUnconnected=off
  wires:
  InputConversion2/1 -> Sum/2
  InputConversion1/1 -> Product/2
  InputConversion/1 -> Product/1
  Sum/1 -> OutputConversion/1
  Product/1 -> Sum/1
  Input/1 -> InputConversion/1, Switch/3
  Switch/1 -> Output/1
  Override_Offset/1 -> InputConversion2/1
  Override_Flag/1 -> Switch/2
  Override_Gain/1 -> InputConversion1/1
  OutputConversion/1 -> Switch/1

== system common_lib/SCond/ramp to zero ==
  note: Common Library::Signal Conditioning::Ramp to Zero
  note: factor is zero at zero speed
      | factor is 1 or -1 if the abs value of spd is > limit
      | factor is linear between 1 and-1 if the abs value of spd < limit
      | the sign of factor is the same as the sign of speed
  speed : Inport
  limit : Inport  Port=2
  Abs : Abs  ZeroCross=off  SaturateOnIntegerOverflow=off
  Constant : Constant  Value=One
  Constant1 : Constant  Value=MinusOne
  Constant2 : Constant  Value=Zero
  Product1 : Product  Inputs=*/  InputSameDT=on  OutDataTypeStr=Inherit: Same as first input
  Relational Operator : RelationalOperator  Operator=<  ZeroCross=off
  Relational Operator1 : RelationalOperator  ZeroCross=off
  Switch : Switch  Threshold=0.5  ZeroCross=off  SaturateOnIntegerOverflow=off
  Switch1 : Switch  Threshold=0.5  ZeroCross=off  SaturateOnIntegerOverflow=off
  factor : Outport  VectorParamsAs1DForOutWhenUnconnected=off
  wires:
  speed/1 -> Abs/1, Relational Operator1/1, Product1/1
  Abs/1 -> Relational Operator/1
  limit/1 -> Product1/2, Relational Operator/2
  Product1/1 -> Switch/1
  Relational Operator/1 -> Switch/2
  Constant/1 -> Switch1/1
  Switch/1 -> factor/1
  Constant1/1 -> Switch1/3
  Constant2/1 -> Relational Operator1/2
  Relational Operator1/1 -> Switch1/2
  Switch1/1 -> Switch/3

== system common_lib/Signal Conditioning/2nd Order Butterworth Filter ==
  note: DO NOT CHANGE 2.0 DAMPING CONSTANT
  note: This is a 2nd order butterworth filter.
      | When Disable is true the raw value is
      | passed through.
  note: The Integrator blocks in common_lib don't work as well
      | for this filter.
  Input : Inport
  CutoffFreq : Inport  Port=2
  Reset : Inport  Port=3
  ClampAboveZero : $bdroot/Misc/ClampAboveZero  Tol=single(0.001)
      settings: AttributesFormatString=tol=%<Tol>
  Constant1 : Constant  Value=single(0.0)  SampleTime=-1
  Constant2 : Constant  Value=single(2.0)  SampleTime=-1
  Constant3 : Constant  Value=TSAMP  SampleTime=-1
  Constant4 : Constant  Value=single(1.0)  SampleTime=-1
  Data Type Conversion : DataTypeConversion  OutDataTypeStr=single  SaturateOnIntegerOverflow=off
  Divide : Product  Inputs=***
  Divide1 : Product  Inputs=***
  Divide2 : Product  Inputs=*/
  ForwardEulerIntergrator1 : MBD_EPS_Local_Blockset/Integrators/ForwardEulerIntergrator  IC=single(0.0)  TSAMP=TSAMP
  ForwardEulerIntergrator2 : MBD_EPS_Local_Blockset/Integrators/ForwardEulerIntergrator  IC=IC  TSAMP=TSAMP
  MinMax : MinMax  Inputs=2  InputSameDT=on  ZeroCross=off
  Sum : Sum  Inputs=|+-
  Sum1 : Sum  Inputs=|+-
  PtmShiftMotorTorqueCmd : Outport  VectorParamsAs1DForOutWhenUnconnected=off
  wires:
  Input/1 -> Sum/1, ForwardEulerIntergrator2/2
  Reset/1 -> ForwardEulerIntergrator2/3, ForwardEulerIntergrator1/3
  ForwardEulerIntergrator1/1 -> Divide1/3, ForwardEulerIntergrator2/1
  Sum1/1 -> ForwardEulerIntergrator1/1
  Divide1/1 -> Sum1/2
  Constant2/1 -> Divide1/2
  Sum/1 -> Divide/1
  ForwardEulerIntergrator2/1 -> PtmShiftMotorTorqueCmd/1, Sum/2
  Divide/1 -> Sum1/1
  Constant1/1 -> ForwardEulerIntergrator1/2
  CutoffFreq/1 -> MinMax/1
  Constant3/1 -> Data Type Conversion/1
  Constant4/1 -> Divide2/1
  Data Type Conversion/1 -> ClampAboveZero/1
  ClampAboveZero/1 -> Divide2/2
  Divide2/1 -> MinMax/2
  MinMax/1 -> [ProtectedCutoffFreq]
  [ProtectedCutoffFreq] -> Divide1/1, Divide/3, Divide/2

== system common_lib/Signal Conditioning/AnalogChecking ==
  in : Inport  OutDataTypeStr=Bus: BO_InputSignal
  u_lim : Inport  Port=2
  l_lim : Inport  Port=3
  r_lim : Inport  Port=4
  tau : Inport  Port=5
  overide : Inport  Port=6
  overide_value : Inport  Port=7
  Bitwise Operator : simulink/Logic and Bit Operations/Bitwise Operator  logicop=OR  UseBitMask=off  NumInputPorts=3  BitMask=bin2dec('11011001')  BitMaskRealWorld=Stored Integer
  Bus Creator2 : BusCreator  Inputs=2  OutDataTypeStr=Bus: BO_InputSignal
  Bus Selector1 : BusSelector  OutputSignals=value,FMI
  C_Calibration1 : Constant  Value=F_OUTOFRANGE
  C_Calibration2 : Constant  Value=F_NOFAULT
  C_Calibration3 : Constant  Value=false
  C_Calibration4 : Constant  Value=F_RATELIMIT
  C_Calibration5 : Constant  Value=F_NOFAULT
  C_Calibration6 : Constant  Value=false
  C_Calibration7 : Constant  Value=F_NOFAULT
  C_Calibration8 : Constant  Value=false
  Fltr_wR : $bdroot/Fltrs/Fltr_wR  TimeStep=TimeStep
  Logical Operator : Logic  Operator=OR
  OOR Fault Detection : $bdroot/Diag/OOR Fault Detection  InitialValue=0
  Rate Limit Fault Detection : $bdroot/Diag/Rate Limit Fault Detection  IC=0  TimeStep=TimeStep
  Relational Operator : RelationalOperator  Operator=~=  OutDataTypeStr=boolean  ZeroCross=off  InputSameDT=off
  Switch : Switch  Threshold=0.5  ZeroCross=off  SaturateOnIntegerOverflow=off  InputSameDT=off
  Switch1 : Switch  Threshold=0.5  ZeroCross=off  SaturateOnIntegerOverflow=off  InputSameDT=off
  Switch2 : Switch  Threshold=0.5  ZeroCross=off  SaturateOnIntegerOverflow=off  InputSameDT=off
  Unit Delay : UnitDelay  InitialCondition=true  SampleTime=-1  HasFrameUpgradeWarning=on
      settings: AttributesFormatString=ic=%<X0>
  out : Outport  VectorParamsAs1DForOutWhenUnconnected=off
  wires:
  Relational Operator/1 -> Logical Operator/2
  Logical Operator/1 -> Fltr_wR/4
  Unit Delay/1 -> Logical Operator/1
  C_Calibration8/1 -> Unit Delay/1
  Bus Selector1/1 -> OOR Fault Detection/1  "<value>"
  C_Calibration6/1 -> OOR Fault Detection/4
  in/1 -> Bus Selector1/1
  OOR Fault Detection/1 -> Rate Limit Fault Detection/1
  u_lim/1 -> OOR Fault Detection/2
  l_lim/1 -> OOR Fault Detection/3
  Bus Selector1/2 -> Bitwise Operator/3  "<FMI>"
  OOR Fault Detection/2 -> Switch/2
  Switch/1 -> Bitwise Operator/2
  C_Calibration1/1 -> Switch/1
  C_Calibration2/1 -> Switch/3
  Bus Creator2/1 -> out/1
  Rate Limit Fault Detection/1 -> Fltr_wR/3, Fltr_wR/1
  r_lim/1 -> Rate Limit Fault Detection/2
  C_Calibration3/1 -> Rate Limit Fault Detection/3
  Rate Limit Fault Detection/2 -> Switch1/2
  C_Calibration4/1 -> Switch1/1
  C_Calibration5/1 -> Switch1/3
  Switch1/1 -> Bitwise Operator/1
  Bitwise Operator/1 -> Bus Creator2/2, Relational Operator/2  "FMI"
  tau/1 -> Fltr_wR/2
  C_Calibration7/1 -> Relational Operator/1
  overide/1 -> Switch2/2
  overide_value/1 -> Switch2/1
  Fltr_wR/1 -> Switch2/3  "value"
  Switch2/1 -> Bus Creator2/1  "value"

== system common_lib/Signal Conditioning/DitherSaturation ==
  signal_in : Inport
  max_signal_amp : Inport  Port=2
  dither_amplitude : Inport  Port=3
  dither_in : Inport  Port=4
  Constant1 : Constant  Value=0  OutDataTypeStr=single
  Constant2 : Constant  Value=single(1)
  Constant3 : Constant  Value=eps  OutDataTypeStr=single
  MinMax1 : MinMax  Inputs=2
  MinMax2 : MinMax  Inputs=2
  MinMax3 : MinMax  Function=max  Inputs=2
  MinMax4 : MinMax  Inputs=2
  MinMax5 : MinMax  Function=max  Inputs=2
  Product : Product  RndMeth=Zero
  Product1 : Product  RndMeth=Zero
  Product2 : Product  Inputs=/*  RndMeth=Zero
  Product3 : Product  Inputs=/*  RndMeth=Zero
  Sum : Sum  Inputs=|-+
  Sum1 : Sum  Inputs=|++
  out : Outport  VectorParamsAs1DForOutWhenUnconnected=off
  wires:
  Constant1/1 -> MinMax5/2
  signal_in/1 -> MinMax5/1
  MinMax5/1 -> MinMax4/2
  MinMax4/1 -> Product2/2, Sum/1, Sum1/2
  Product1/1 -> Sum1/1
  Sum1/1 -> out/1
  dither_in/1 -> Product/1
  MinMax3/1 -> Product2/1, Product3/1
  Constant3/1 -> MinMax3/2
  Product/1 -> Product1/1
  Product3/1 -> MinMax1/2
  Sum/1 -> Product3/2
  Product2/1 -> MinMax1/1
  MinMax2/1 -> Product1/2
  MinMax1/1 -> MinMax2/2
  Constant2/1 -> MinMax2/1
  max_signal_amp/1 -> MinMax4/1, Sum/2
  dither_amplitude/1 -> Product/2, MinMax3/1

== system common_lib/Signal Conditioning/DitherSaturation1 ==
  signal_in : Inport
  max_signal_amp : Inport  Port=2
  dither_amplitude : Inport  Port=3
  dither_in : Inport  Port=4
  Constant1 : Constant  Value=0  OutDataTypeStr=single
  Constant2 : Constant  Value=single(1)
  Constant3 : Constant  Value=eps  OutDataTypeStr=single
  MinMax1 : MinMax  Inputs=2
  MinMax2 : MinMax  Inputs=2
  MinMax3 : MinMax  Function=max  Inputs=2
  MinMax4 : MinMax  Inputs=2
  MinMax5 : MinMax  Function=max  Inputs=2
  Product : Product  RndMeth=Zero
  Product1 : Product  RndMeth=Zero
  Product2 : Product  Inputs=/*  RndMeth=Zero
  Product3 : Product  Inputs=/*  RndMeth=Zero
  Sum : Sum  Inputs=|-+
  Sum1 : Sum  Inputs=|++
  out : Outport  VectorParamsAs1DForOutWhenUnconnected=off
  wires:
  Constant1/1 -> MinMax5/2
  signal_in/1 -> MinMax5/1
  MinMax5/1 -> MinMax4/2
  MinMax4/1 -> Product2/2, Sum/1, Sum1/2
  Product1/1 -> Sum1/1
  Sum1/1 -> out/1
  dither_in/1 -> Product/1
  MinMax3/1 -> Product2/1, Product3/1
  Constant3/1 -> MinMax3/2
  Product/1 -> Product1/1
  Product3/1 -> MinMax1/2
  Sum/1 -> Product3/2
  Product2/1 -> MinMax1/1
  MinMax2/1 -> Product1/2
  MinMax1/1 -> MinMax2/2
  Constant2/1 -> MinMax2/1
  max_signal_amp/1 -> MinMax4/1, Sum/2
  dither_amplitude/1 -> Product/2, MinMax3/1

== system common_lib/Signal Conditioning/HydValveDither ==
  freq_hz : Inport
  CalculateActualFreq : Subsystem
  Constant : Constant  Value=single(ts)
  Constant4 : Constant  Value=single(0)
  Switch : Switch  Criteria=u2 > Threshold  SaturateOnIntegerOverflow=off  InputSameDT=off
  TableBasedSignalGen : Subsystem
  out : Outport  VectorParamsAs1DForOutWhenUnconnected=off
  realized_freq : Outport  Port=2  VectorParamsAs1DForOutWhenUnconnected=off
  wires:
  Constant4/1 -> Switch/3
  TableBasedSignalGen/1(out) -> Switch/1
  freq_hz/1 -> CalculateActualFreq/1(desired_freqency_hz), Switch/2
  CalculateActualFreq/2(sample_times_per_cycle) -> TableBasedSignalGen/1(sample_times_per_cycle)
  CalculateActualFreq/1(realized_freq) -> realized_freq/1
  Constant/1 -> CalculateActualFreq/2(sample_time)
  Switch/1 -> out/1
